simulink model "FDCDC_PSS_40msdelay_Github"  (R2016a)
settings: Solver=ode23t  StartTime=0  StopTime=10  MaxStep=1e-1  RelTol=1e-3
undefined symbols (not defined in the file): D1, delayM2, Delta
libraries: powerlib x29, sps_avr x3, truetime x3, fuzblock x1, spsExcitationSystemModel x1
settings Model: Creator=Administrator  LastModifiedBy=85323
settings SolverCC: SolverResetMethod=Robust
settings DataIOCC: LimitDataPoints=on  SaveFormat=Array
settings HardwareCC: ProdBitPerPointer=32  ProdLargestAtomicFloat=None  ProdIntDivRoundTo=Undefined  ProdEndianess=Unspecified  ProdWordSize=32  ProdHWDeviceType=32-bit Generic
settings ModelReferenceCC: PropagateSignalLabelsOutOfModel=off
settings ConfigComp: CovModelRefEnable=Off

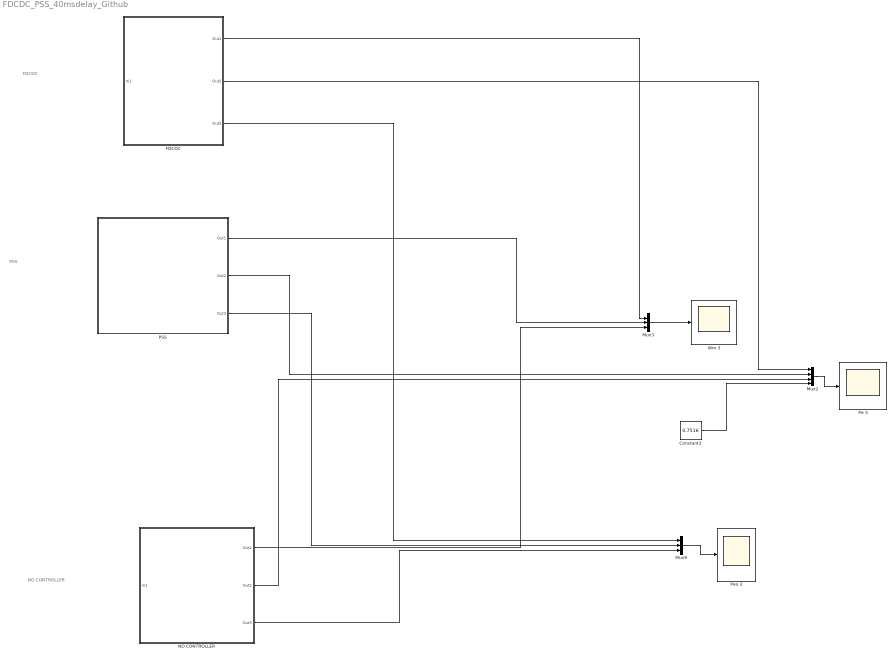
== system FDCDC_PSS_40msdelay_Github ==
  note: PSS
  note: NO
      | CONTROLLER
  note: FDCDC
  Constant3 : Constant  Value=0.7516
  FDCDC : Subsystem
  Mux2 : Mux
  Mux3 : Mux  Inputs=3
  Mux9 : Mux  Inputs=3
  NO CONTROLLER : Subsystem
  PSS : Subsystem
  Pe 3 : Scope
  Peo 3 : Scope
  Wm 3 : Scope
  wires:
  Mux9/1 -> Peo 3/1
  Mux3/1 -> Wm 3/1
  Mux2/1 -> Pe 3/1
  FDCDC/1(Out1) -> Mux3/1
  FDCDC/2(Out2) -> Mux2/1
  FDCDC/3(Out3) -> Mux9/1
  PSS/1(Out1) -> Mux3/2
  PSS/2(Out2) -> Mux2/2
  PSS/3(Out3) -> Mux9/2
  NO CONTROLLER/1(Out1) -> Mux3/3
  NO CONTROLLER/2(Out2) -> Mux2/3
  NO CONTROLLER/3(Out3) -> Mux9/3
  Constant3/1 -> Mux2/4

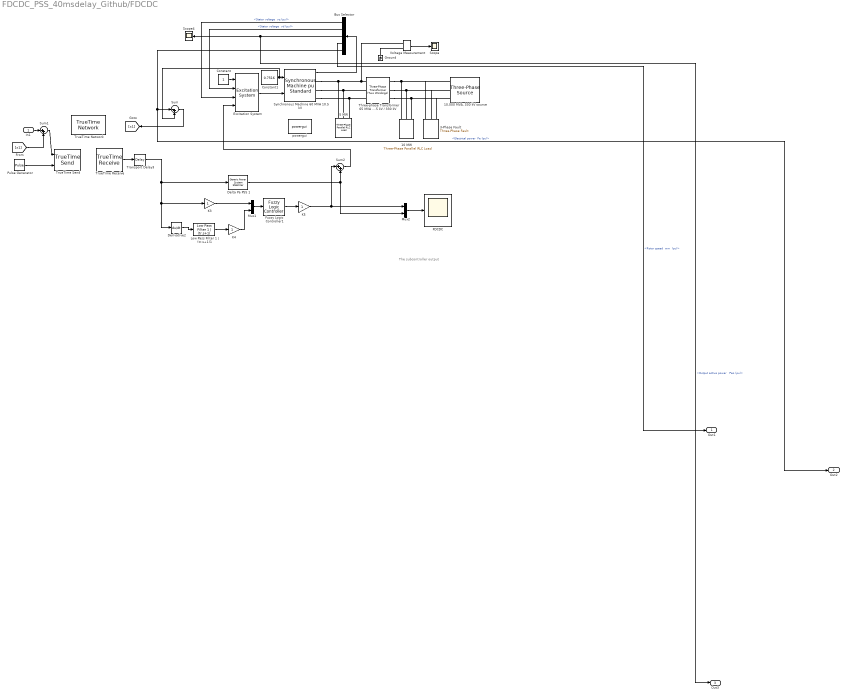
== system FDCDC_PSS_40msdelay_Github/FDCDC ==
  note: The subcontroller output
  In1 : Inport
  10 MW : powerlib/Elements/Three-Phase Parallel RLC Load  LConnTagsString=A|B|C  Configuration=Y (grounded)  NominalVoltage=230e3  Vabc=[1e3 1e3 1e3]  Vabcp=[1e3 1e3 1e3]  NominalFrequency=60  UnbalancedPower=off  ActivePower=10000000  InductivePower=0  CapacitivePower=0  Pabc=[10e3 9e3 11e3]  QLabc=[100 90 110]  QCabc=[100 90 110]  Pabcp=[10e3 9e3 11e3]  QLabcp=[100 90 110]  QCabcp=[100 90 110]  Measurements=None  LoadType=constant Z
  "10,000 MVA, 330 kV source" : powerlib/Electrical Sources/Three-Phase Source  InternalConnection=Yg  VoltagePhases=off  Voltage=(330000)*1.00006  PhaseAngle=-0.77547  Voltage_phases=[25e3 25e3 25e3]/sqrt(3)  PhaseAngles_phases=[0 -120 +120]  Frequency=50  NonIdealSource=on  SpecifyImpedance=on  Resistance=0.529  Inductance=0.0140  ShortCircuitLevel=10000e6  BaseVoltage=230e3  XRratio=10  BusType=swing  Pref=0  Qref=0  Prefabc=[10e3, 10e3, 10e3]  Qrefabc=[0, 0, 0]  Qmin=-Inf  Qmax=Inf
  3-Phase Fault : powerlib/Elements/Three-Phase Fault  InitialStates=0  FaultA=on  FaultB=on  FaultC=on  GroundFault=on  SwitchTimes=[ 2 2.2]  External=off  SwitchStatus=NaN  FaultResistance=1e-3  GroundResistance=1e-3  SnubberResistance=inf  SnubberCapacitance=inf  Measurements=None
  5 MW : powerlib/Elements/Three-Phase Parallel RLC Load  LConnTagsString=A|B|C  Configuration=Y (grounded)  NominalVoltage=13.8e3  Vabc=[1e3 1e3 1e3]  Vabcp=[1e3 1e3 1e3]  NominalFrequency=60  UnbalancedPower=off  ActivePower=5000000  InductivePower=0  CapacitivePower=0  Pabc=[10e3 9e3 11e3]  QLabc=[100 90 110]  QCabc=[100 90 110]  Pabcp=[10e3 9e3 11e3]  QLabcp=[100 90 110]  QCabcp=[100 90 110]  Measurements=None  LoadType=constant Z
  Bus Selector : BusSelector  OutputSignals="dq0 components.Stator voltage  vq (pu),dq0 components.Stator voltage  vd (pu),Output active power   Peo (pu),Mechanical.Rotor speed  wm  (pu),Mechanical.Electrical power  Pe (pu)"
  Constant : Constant
  Constant1 : Constant  Value=0.7516
  Delta Pa PSS 1 : powerlib/Machines/Generic Power System Stabilizer  Tsensor=15e-3  K=2.5*1.25  Twashout=1  Tleadlag1=[60e-3 1]  Tleadlag2=[0 0]  VSlimits=[-1 1]  Vinit=0  Plot_On=off  MagdB_On=off  FreqRange=logspace(-2,2,500)
  Derivative2 : Derivative
  Excitation System : sps_avr/Excitation System  tr=20e-3  reg=[ 300, 0.001 ]  exc=[ 1, 0 ]  tgr=[ 0, 0 ]  damp=[ 0.001, 0.1 ]  sat=[ 0, 0 ]  lim=[ -11.5, 11.5, 0 ]  v0=[1,1.29071]
  FDCDC : Scope
  Fuzzy Logic Controller1 : fuzblock/Fuzzy Logic  Controller  fis=[delayM2]
  Ground : powerlib/Elements/Ground  LConnTagsString=a
  K3 : Gain
  K4 : Gain
  K5 : Gain
  Low Pass Filter 1 | (tr.s+1)1 : spsExcitationSystemModel/Continuous/Low Pass Filter 1 | (tr.s+1)  N=1  D=[0.2 1]  Y0=0  U0=0
  Mux1 : Mux  Inputs=2
  Mux2 : Mux  Inputs=2
  Pulse Generator : DiscretePulseGenerator  PulseType=Time based  Period=0.01  PulseWidth=80
  Scope : Scope
  Scope4 : Scope
  Sum : Sum  Inputs=|-+
  Sum1 : Sum  Inputs=|++
  Sum2 : Sum  Inputs=|++
  Synchronous Machine 60 MVA 10.5 kV : powerlib/Machines/Synchronous Machine pu Standard  PresetModel=No  MechanicalLoad=Mechanical power Pm  ShowDetailedParameters=on  RotorType=Salient-pole  Units=per unit standard parameters  MeasurementBus=off  NominalParameters="[ 60E6  10500   50 ]"  Reactances1=[ 31 32 33 34 35 36 37 ]  Reactances2=[ 1.305, 0.296, 0.252, 0.474, 0.243, 0.18 ]  dAxisTimeConstants=Short-circuit  qAxisTimeConstants=Open-circuit  TimeConstants1=[]  TimeConstants2=[]  TimeConstants3=[]  TimeConstants4=[]  TimeConstants5=[ 1.01, 0.053, 0.1 ]  TimeConstants6=[]  TimeConstants7=[]  TimeConstants8=[]  StatorResistance=2.8544e-3  Mechanical=[ 3.2 0 2]  PolePairs=2  InitialConditions=[0 -94.2826 0.750185 0.750185 0.750185 -24.943 -144.943 95.057 1.29071]  SetSaturation=off  Saturation=[0.6404,0.7127,0.8441,0.9214,0.9956,1.082,1.19,1.316,1.457;0.7,0.7698,0.8872,0.9466,0.9969,1.046,1.1,1.151,1.201]  LoadFlowParameters=[1 150000000 0 0]  TsPowergui=0  TsBlock=-1  IterativeModel=Trapezoidal non iterative  IterativeDiscreteModel=Trapezoidal non iterative  BusType=PV  Pref=150000000  Qref=0  Qmin=-Inf  Qmax=Inf  PLF=0  QLF=0
      settings: AttributesFormatString=\n\n
  Three-phase Transformer 65 MVA 10.5 kV / 330 kV : powerlib/Elements/Three-Phase Transformer (Two Windings)  Winding1Connection=Delta (D1)  Winding2Connection=Yg  CoreType=Three single-phase transformers  SetSaturation=off  Hysteresis=off  DataFile='hysteresis'  SetInitialFlux=off  Measurements=None  UNITS=pu  NominalPower=[ 65e6 50 ]  Winding1="[ 10.5e3 0.0027  0.08]"  Winding2=[ 330e3 0.0027 0.08]  Rm=500  Lm=500  L0=0.5  Saturation="[ 0,0  ;  0.005,1.2  ;  1.0,1.4 ]"  InitialFluxes=[ 0.8 , -0.8 , 0.7 ]  MoreParameters=off  BreakLoop=off  DataType=off  TransfoNumber=0
  Transport Delay3 : TransportDelay  DelayTime=0.04
  TrueTime Network : truetime/TrueTime Network  nwtype=CSMA/CD (Ethernet)  nwnbr=1  nnodes=1  rate=10000000  minsize=512  lossprob=0  seed=0  bandwidths=[0.5 0.5]  slotsize=512  schedule=[1 1 2]  memsize=80000  buftype=Common buffer  overflow=Retransmit  dynSchedule=0  miniSlotSize=0  NIT=0  QSortMode=FIFO  sync=0  irtSchedule=0  nrtLength=0  nodeGraph=0  scheduleoutput=off
  TrueTime Receive : truetime/TrueTime Receive  nwnbr=1  receiver=1  outdim=1  triggeroutput=off  senderoutput=off  lengthoutput=off  priorityoutput=off  timestampoutput=off  signalpoweroutput=off  msgIDoutput=off
  TrueTime Send : truetime/TrueTime Send  trigger=falling  nwnbr=1  sender=1  indim=1  recsource=internal  receiver=1  lengthsource=internal  length=1000  priosource=internal  prio=1  msgIDsource=internal  msgID=0  dynamicSegment=dynamic
  Voltage Measurement : powerlib/Measurements/Voltage Measurement  PhasorSimulation=off  OutputType=Complex  PSBequivalent=0
  powergui : powerlib/powergui  Priority=1  SimulationMode=Continuous  SolverType=Tustin/Backward Euler (TBE)  SampleTime=1e-6  frequency=60  SPID=off  DisableSnubberDevices=off  DisableRonSwitches=off  DisableVfSwitches=off  SwTol=0  DisplayEquations=off  Interpol=off  ExternalGateDelay=off  methode=off  Ts=100  FunctionMessages=off  echomessages=off  HookPort=off  EnableUseOfTLC=off  x0status=blocks  frequencyindice=50  Pbase=100e6  ErrMax=1e-4  Iterations=50  UnitsV=kV  UnitsW=MW  buscounter=0  RestoreLinks=warning  ResistiveCurrentMeasurement=off  Frange=[0:2:500]  Ylog=off  Xlog=on  ShowGrid=off  save=off  variable=ZData  structure=0  ZoomFFT=off  StartTime=0.0  cycles=1  DisplayStyle=1  fundamental=60  FreqAxis=off  MaxFrequency=1000  frequencyindicesteady=1  RmsSteady=1  display=off
  Out1 : Outport
  Out2 : Outport  Port=2
  Out3 : Outport  Port=3
  wires:
  In1/1 -> Sum1/1
  Sum1/1 -> TrueTime Send/1
  Bus Selector/1 -> Excitation System/3  "<Stator voltage  vq (pu)>"
  Pulse Generator/1 -> TrueTime Send/2
  [x1] -> Sum1/2
  Synchronous Machine 60 MVA 10.5 kV/1 -> Bus Selector/1
  Constant/1 -> Excitation System/1
  Bus Selector/3 -> Out3/1, Scope4/1  "<Output active power   Peo (pu)>"
  Bus Selector/5 -> Out2/1, Sum/1  "<Electrical power  Pe (pu)>"
  Voltage Measurement/1 -> Scope/1
  Mux1/1 -> Fuzzy Logic Controller1/1
  K4/1 -> Mux1/2
  Sum/1 -> [x1]
  Derivative2/1 -> Low Pass Filter 1 | (tr.s+1)1/1
  Sum2/1 -> Excitation System/4
  TrueTime Receive/1 -> Transport Delay3/1
  Fuzzy Logic Controller1/1 -> K5/1
  Constant1/1 -> Sum/2, Synchronous Machine 60 MVA 10.5 kV/1
  K3/1 -> Mux1/1
  K5/1 -> Sum2/1, Mux2/1
  Low Pass Filter 1 | (tr.s+1)1/1 -> K4/1
  Transport Delay3/1 -> Delta Pa PSS 1/1, K3/1, Derivative2/1
  Bus Selector/2 -> Excitation System/2  "<Stator voltage  vd (pu)>"
  Bus Selector/4 -> Out1/1  "<Rotor speed  wm  (pu)>"
  Excitation System/1 -> Synchronous Machine 60 MVA 10.5 kV/2
  Delta Pa PSS 1/1 -> Mux2/2, Sum2/2
  Mux2/1 -> FDCDC/1
  connections:
  Voltage Measurement/LConn2 -- Ground/LConn1
  Synchronous Machine 60 MVA 10.5 kV/RConn3 -- Three-phase Transformer 65 MVA 10.5 kV / 330 kV/LConn3 -- 5 MW/LConn3
  Synchronous Machine 60 MVA 10.5 kV/RConn2 -- Three-phase Transformer 65 MVA 10.5 kV / 330 kV/LConn2 -- 5 MW/LConn2
  Three-phase Transformer 65 MVA 10.5 kV / 330 kV/RConn3 -- "10,000 MVA, 330 kV source"/RConn3 -- 3-Phase Fault/LConn3 -- 10 MW/LConn3
  Three-phase Transformer 65 MVA 10.5 kV / 330 kV/RConn1 -- "10,000 MVA, 330 kV source"/RConn1 -- 3-Phase Fault/LConn1 -- 10 MW/LConn1
  Voltage Measurement/LConn1 -- Three-phase Transformer 65 MVA 10.5 kV / 330 kV/LConn1 -- Synchronous Machine 60 MVA 10.5 kV/RConn1 -- 5 MW/LConn1
  Three-phase Transformer 65 MVA 10.5 kV / 330 kV/RConn2 -- "10,000 MVA, 330 kV source"/RConn2 -- 3-Phase Fault/LConn2 -- 10 MW/LConn2

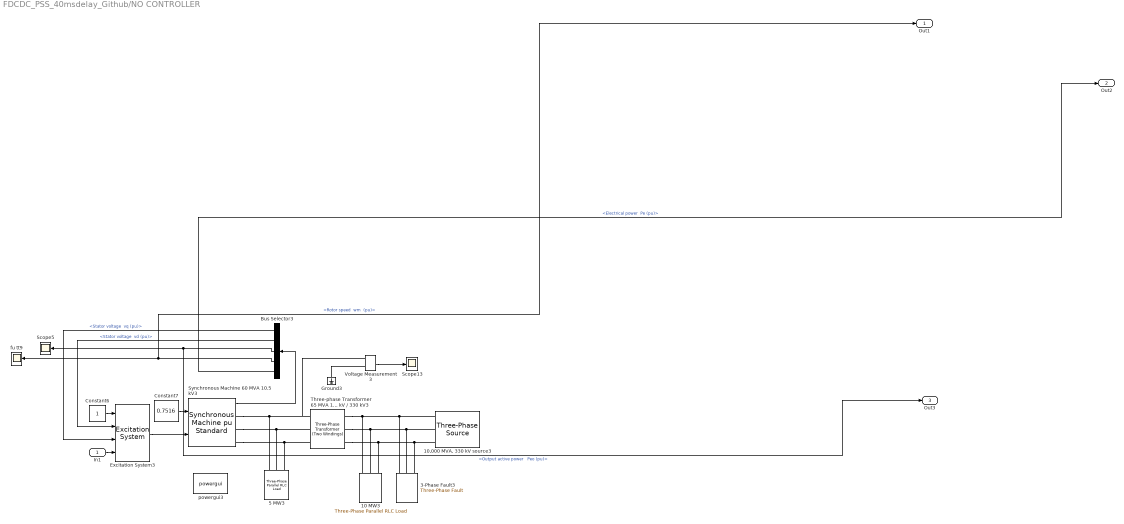
== system FDCDC_PSS_40msdelay_Github/NO CONTROLLER ==
  In1 : Inport
  10 MW3 : powerlib/Elements/Three-Phase Parallel RLC Load  LConnTagsString=A|B|C  Configuration=Y (grounded)  NominalVoltage=230e3  Vabc=[1e3 1e3 1e3]  Vabcp=[1e3 1e3 1e3]  NominalFrequency=60  UnbalancedPower=off  ActivePower=10000000  InductivePower=0  CapacitivePower=0  Pabc=[10e3 9e3 11e3]  QLabc=[100 90 110]  QCabc=[100 90 110]  Pabcp=[10e3 9e3 11e3]  QLabcp=[100 90 110]  QCabcp=[100 90 110]  Measurements=None  LoadType=constant Z
  "10,000 MVA, 330 kV source3" : powerlib/Electrical Sources/Three-Phase Source  InternalConnection=Yg  VoltagePhases=off  Voltage=(330000)*1.00006  PhaseAngle=-0.77547  Voltage_phases=[25e3 25e3 25e3]/sqrt(3)  PhaseAngles_phases=[0 -120 +120]  Frequency=50  NonIdealSource=on  SpecifyImpedance=on  Resistance=0.529  Inductance=0.0140  ShortCircuitLevel=10000e6  BaseVoltage=230e3  XRratio=10  BusType=swing  Pref=0  Qref=0  Prefabc=[10e3, 10e3, 10e3]  Qrefabc=[0, 0, 0]  Qmin=-Inf  Qmax=Inf
  3-Phase Fault3 : powerlib/Elements/Three-Phase Fault  InitialStates=0  FaultA=on  FaultB=on  FaultC=on  GroundFault=on  SwitchTimes=[2 2.2]  External=off  SwitchStatus=NaN  FaultResistance=1e-3  GroundResistance=1e-3  SnubberResistance=inf  SnubberCapacitance=inf  Measurements=None
  5 MW3 : powerlib/Elements/Three-Phase Parallel RLC Load  LConnTagsString=A|B|C  Configuration=Y (grounded)  NominalVoltage=13.8e3  Vabc=[1e3 1e3 1e3]  Vabcp=[1e3 1e3 1e3]  NominalFrequency=60  UnbalancedPower=off  ActivePower=5000000  InductivePower=0  CapacitivePower=0  Pabc=[10e3 9e3 11e3]  QLabc=[100 90 110]  QCabc=[100 90 110]  Pabcp=[10e3 9e3 11e3]  QLabcp=[100 90 110]  QCabcp=[100 90 110]  Measurements=None  LoadType=constant Z
  Bus Selector3 : BusSelector  OutputSignals="dq0 components.Stator voltage  vq (pu),dq0 components.Stator voltage  vd (pu),Output active power   Peo (pu),Mechanical.Rotor speed  wm  (pu),Mechanical.Electrical power  Pe (pu)"
  Constant6 : Constant
  Constant7 : Constant  Value=0.7516
  Excitation System3 : sps_avr/Excitation System  tr=20e-3  reg=[ 300, 0.001 ]  exc=[ 1, 0 ]  tgr=[ 0, 0 ]  damp=[ 0.001, 0.1 ]  sat=[ 0, 0 ]  lim=[ -11.5, 11.5, 0 ]  v0=[1,1.29071]
  Ground3 : powerlib/Elements/Ground  LConnTagsString=a
  Scope13 : Scope
  Scope5 : Scope
  Synchronous Machine 60 MVA 10.5 kV3 : powerlib/Machines/Synchronous Machine pu Standard  PresetModel=No  MechanicalLoad=Mechanical power Pm  ShowDetailedParameters=on  RotorType=Salient-pole  Units=per unit standard parameters  MeasurementBus=off  NominalParameters="[ 60E6  10500   50 ]"  Reactances1=[ 31 32 33 34 35 36 37 ]  Reactances2=[ 1.305, 0.296, 0.252, 0.474, 0.243, 0.18 ]  dAxisTimeConstants=Short-circuit  qAxisTimeConstants=Open-circuit  TimeConstants1=[]  TimeConstants2=[]  TimeConstants3=[]  TimeConstants4=[]  TimeConstants5=[ 1.01, 0.053, 0.1 ]  TimeConstants6=[]  TimeConstants7=[]  TimeConstants8=[]  StatorResistance=2.8544e-3  Mechanical=[ 3.2 0 2]  PolePairs=2  InitialConditions=[0 -94.2826 0.750185 0.750185 0.750185 -24.943 -144.943 95.057 1.29071]  SetSaturation=off  Saturation=[0.6404,0.7127,0.8441,0.9214,0.9956,1.082,1.19,1.316,1.457;0.7,0.7698,0.8872,0.9466,0.9969,1.046,1.1,1.151,1.201]  LoadFlowParameters=[1 150000000 0 0]  TsPowergui=0  TsBlock=-1  IterativeModel=Trapezoidal non iterative  IterativeDiscreteModel=Trapezoidal non iterative  BusType=PV  Pref=150000000  Qref=0  Qmin=-Inf  Qmax=Inf  PLF=0  QLF=0
      settings: AttributesFormatString=\n\n
  Three-phase Transformer 65 MVA 10.5 kV / 330 kV3 : powerlib/Elements/Three-Phase Transformer (Two Windings)  Winding1Connection=Delta (D1)  Winding2Connection=Yg  CoreType=Three single-phase transformers  SetSaturation=off  Hysteresis=off  DataFile='hysteresis'  SetInitialFlux=off  Measurements=None  UNITS=pu  NominalPower=[ 65e6 50 ]  Winding1="[ 10.5e3 0.0027  0.08]"  Winding2=[ 330e3 0.0027 0.08]  Rm=500  Lm=500  L0=0.5  Saturation="[ 0,0  ;  0.005,1.2  ;  1.0,1.4 ]"  InitialFluxes=[ 0.8 , -0.8 , 0.7 ]  MoreParameters=off  BreakLoop=off  DataType=off  TransfoNumber=0
  Voltage Measurement3 : powerlib/Measurements/Voltage Measurement  PhasorSimulation=off  OutputType=Complex  PSBequivalent=0
  fu tt9 : Scope
  powergui3 : powerlib/powergui  Priority=1  SimulationMode=Continuous  SolverType=Tustin/Backward Euler (TBE)  SampleTime=1e-6  frequency=60  SPID=off  DisableSnubberDevices=off  DisableRonSwitches=off  DisableVfSwitches=off  SwTol=0  DisplayEquations=off  Interpol=off  ExternalGateDelay=off  methode=off  Ts=100  FunctionMessages=off  echomessages=off  HookPort=off  EnableUseOfTLC=off  x0status=blocks  frequencyindice=50  Pbase=100e6  ErrMax=1e-4  Iterations=50  UnitsV=kV  UnitsW=MW  buscounter=0  RestoreLinks=warning  ResistiveCurrentMeasurement=off  Frange=[0:2:500]  Ylog=off  Xlog=on  ShowGrid=off  save=off  variable=ZData  structure=0  ZoomFFT=off  StartTime=0.0  cycles=1  DisplayStyle=1  fundamental=60  FreqAxis=off  MaxFrequency=1000  frequencyindicesteady=1  RmsSteady=1  display=off
  Out1 : Outport
  Out2 : Outport  Port=2
  Out3 : Outport  Port=3
  wires:
  Bus Selector3/5 -> Out2/1  "<Electrical power  Pe (pu)>"
  Bus Selector3/3 -> Out3/1, Scope5/1  "<Output active power   Peo (pu)>"
  Constant7/1 -> Synchronous Machine 60 MVA 10.5 kV3/1
  Synchronous Machine 60 MVA 10.5 kV3/1 -> Bus Selector3/1
  Voltage Measurement3/1 -> Scope13/1
  Bus Selector3/4 -> Out1/1, fu tt9/1  "<Rotor speed  wm  (pu)>"
  Bus Selector3/2 -> Excitation System3/2  "<Stator voltage  vd (pu)>"
  Constant6/1 -> Excitation System3/1
  Excitation System3/1 -> Synchronous Machine 60 MVA 10.5 kV3/2
  Bus Selector3/1 -> Excitation System3/3  "<Stator voltage  vq (pu)>"
  In1/1 -> Excitation System3/4
  connections:
  Three-phase Transformer 65 MVA 10.5 kV / 330 kV3/LConn3 -- 5 MW3/LConn3 -- Synchronous Machine 60 MVA 10.5 kV3/RConn3
  3-Phase Fault3/LConn3 -- "10,000 MVA, 330 kV source3"/RConn3 -- 10 MW3/LConn3 -- Three-phase Transformer 65 MVA 10.5 kV / 330 kV3/RConn3
  3-Phase Fault3/LConn2 -- "10,000 MVA, 330 kV source3"/RConn2 -- 10 MW3/LConn2 -- Three-phase Transformer 65 MVA 10.5 kV / 330 kV3/RConn2
  3-Phase Fault3/LConn1 -- "10,000 MVA, 330 kV source3"/RConn1 -- 10 MW3/LConn1 -- Three-phase Transformer 65 MVA 10.5 kV / 330 kV3/RConn1
  Three-phase Transformer 65 MVA 10.5 kV / 330 kV3/LConn2 -- 5 MW3/LConn2 -- Synchronous Machine 60 MVA 10.5 kV3/RConn2
  Voltage Measurement3/LConn2 -- Ground3/LConn1
  5 MW3/LConn1 -- Synchronous Machine 60 MVA 10.5 kV3/RConn1 -- Three-phase Transformer 65 MVA 10.5 kV / 330 kV3/LConn1 -- Voltage Measurement3/LConn1

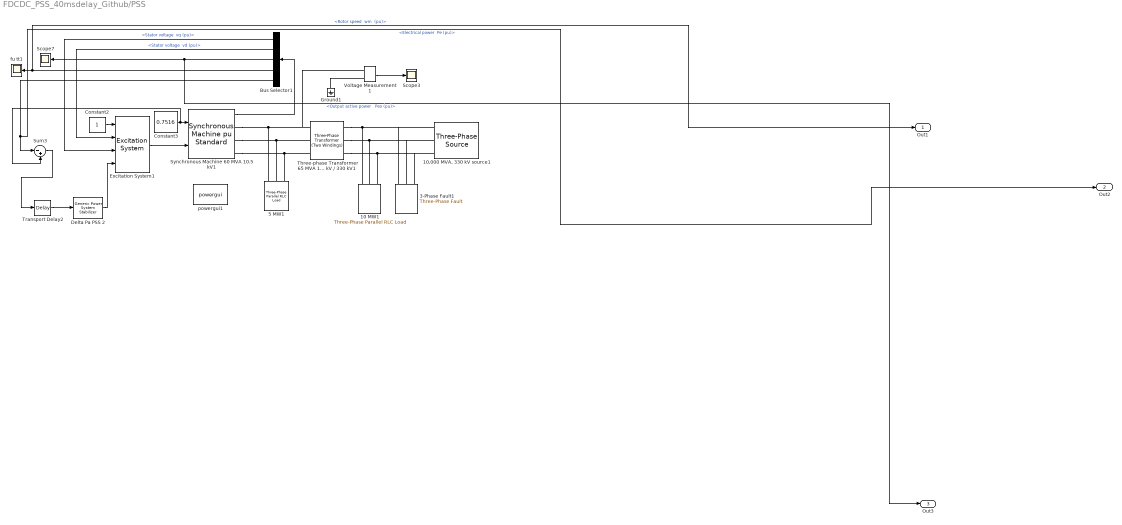
== system FDCDC_PSS_40msdelay_Github/PSS ==
  10 MW1 : powerlib/Elements/Three-Phase Parallel RLC Load  LConnTagsString=A|B|C  Configuration=Y (grounded)  NominalVoltage=230e3  Vabc=[1e3 1e3 1e3]  Vabcp=[1e3 1e3 1e3]  NominalFrequency=60  UnbalancedPower=off  ActivePower=10000000  InductivePower=0  CapacitivePower=0  Pabc=[10e3 9e3 11e3]  QLabc=[100 90 110]  QCabc=[100 90 110]  Pabcp=[10e3 9e3 11e3]  QLabcp=[100 90 110]  QCabcp=[100 90 110]  Measurements=None  LoadType=constant Z
  "10,000 MVA, 330 kV source1" : powerlib/Electrical Sources/Three-Phase Source  InternalConnection=Yg  VoltagePhases=off  Voltage=(330000)*1.00006  PhaseAngle=-0.77547  Voltage_phases=[25e3 25e3 25e3]/sqrt(3)  PhaseAngles_phases=[0 -120 +120]  Frequency=50  NonIdealSource=on  SpecifyImpedance=on  Resistance=0.529  Inductance=0.0140  ShortCircuitLevel=10000e6  BaseVoltage=230e3  XRratio=10  BusType=swing  Pref=0  Qref=0  Prefabc=[10e3, 10e3, 10e3]  Qrefabc=[0, 0, 0]  Qmin=-Inf  Qmax=Inf
  3-Phase Fault1 : powerlib/Elements/Three-Phase Fault  InitialStates=0  FaultA=on  FaultB=on  FaultC=on  GroundFault=on  SwitchTimes=[ 2 2.2]  External=off  SwitchStatus=NaN  FaultResistance=1e-3  GroundResistance=1e-3  SnubberResistance=inf  SnubberCapacitance=inf  Measurements=None
  5 MW1 : powerlib/Elements/Three-Phase Parallel RLC Load  LConnTagsString=A|B|C  Configuration=Y (grounded)  NominalVoltage=13.8e3  Vabc=[1e3 1e3 1e3]  Vabcp=[1e3 1e3 1e3]  NominalFrequency=60  UnbalancedPower=off  ActivePower=5000000  InductivePower=0  CapacitivePower=0  Pabc=[10e3 9e3 11e3]  QLabc=[100 90 110]  QCabc=[100 90 110]  Pabcp=[10e3 9e3 11e3]  QLabcp=[100 90 110]  QCabcp=[100 90 110]  Measurements=None  LoadType=constant Z
  Bus Selector1 : BusSelector  OutputSignals="dq0 components.Stator voltage  vq (pu),dq0 components.Stator voltage  vd (pu),Output active power   Peo (pu),Mechanical.Rotor speed  wm  (pu),Mechanical.Electrical power  Pe (pu)"
  Constant2 : Constant
  Constant3 : Constant  Value=0.7516
  Delta Pa PSS 2 : powerlib/Machines/Generic Power System Stabilizer  Tsensor=15e-3  K=2.5*1.25  Twashout=1  Tleadlag1=[60e-3 1]  Tleadlag2=[0 0]  VSlimits=[-1 1]  Vinit=0  Plot_On=off  MagdB_On=off  FreqRange=logspace(-2,2,500)
  Excitation System1 : sps_avr/Excitation System  tr=20e-3  reg=[ 300, 0.001 ]  exc=[ 1, 0 ]  tgr=[ 0, 0 ]  damp=[ 0.001, 0.1 ]  sat=[ 0, 0 ]  lim=[ -11.5, 11.5, 0 ]  v0=[1,1.29071]
  Ground1 : powerlib/Elements/Ground  LConnTagsString=a
  Scope3 : Scope
  Scope7 : Scope
  Sum3 : Sum  Inputs=|-+
  Synchronous Machine 60 MVA 10.5 kV1 : powerlib/Machines/Synchronous Machine pu Standard  PresetModel=No  MechanicalLoad=Mechanical power Pm  ShowDetailedParameters=on  RotorType=Salient-pole  Units=per unit standard parameters  MeasurementBus=off  NominalParameters="[ 60E6  10500   50 ]"  Reactances1=[ 31 32 33 34 35 36 37 ]  Reactances2=[ 1.305, 0.296, 0.252, 0.474, 0.243, 0.18 ]  dAxisTimeConstants=Short-circuit  qAxisTimeConstants=Open-circuit  TimeConstants1=[]  TimeConstants2=[]  TimeConstants3=[]  TimeConstants4=[]  TimeConstants5=[ 1.01, 0.053, 0.1 ]  TimeConstants6=[]  TimeConstants7=[]  TimeConstants8=[]  StatorResistance=2.8544e-3  Mechanical=[ 3.2 0 2]  PolePairs=2  InitialConditions=[0 -94.2826 0.750185 0.750185 0.750185 -24.943 -144.943 95.057 1.29071]  SetSaturation=off  Saturation=[0.6404,0.7127,0.8441,0.9214,0.9956,1.082,1.19,1.316,1.457;0.7,0.7698,0.8872,0.9466,0.9969,1.046,1.1,1.151,1.201]  LoadFlowParameters=[1 150000000 0 0]  TsPowergui=0  TsBlock=-1  IterativeModel=Trapezoidal non iterative  IterativeDiscreteModel=Trapezoidal non iterative  BusType=PV  Pref=150000000  Qref=0  Qmin=-Inf  Qmax=Inf  PLF=0  QLF=0
      settings: AttributesFormatString=\n\n
  Three-phase Transformer 65 MVA 10.5 kV / 330 kV1 : powerlib/Elements/Three-Phase Transformer (Two Windings)  Winding1Connection=Delta (D1)  Winding2Connection=Yg  CoreType=Three single-phase transformers  SetSaturation=off  Hysteresis=off  DataFile='hysteresis'  SetInitialFlux=off  Measurements=None  UNITS=pu  NominalPower=[ 65e6 50 ]  Winding1="[ 10.5e3 0.0027  0.08]"  Winding2=[ 330e3 0.0027 0.08]  Rm=500  Lm=500  L0=0.5  Saturation="[ 0,0  ;  0.005,1.2  ;  1.0,1.4 ]"  InitialFluxes=[ 0.8 , -0.8 , 0.7 ]  MoreParameters=off  BreakLoop=off  DataType=off  TransfoNumber=0
  Transport Delay2 : TransportDelay  DelayTime=0.04
  Voltage Measurement1 : powerlib/Measurements/Voltage Measurement  PhasorSimulation=off  OutputType=Complex  PSBequivalent=0
  fu tt1 : Scope
  powergui1 : powerlib/powergui  Priority=1  SimulationMode=Continuous  SolverType=Tustin/Backward Euler (TBE)  SampleTime=1e-6  frequency=60  SPID=off  DisableSnubberDevices=off  DisableRonSwitches=off  DisableVfSwitches=off  SwTol=0  DisplayEquations=off  Interpol=off  ExternalGateDelay=off  methode=off  Ts=100  FunctionMessages=off  echomessages=off  HookPort=off  EnableUseOfTLC=off  x0status=blocks  frequencyindice=50  Pbase=100e6  ErrMax=1e-4  Iterations=50  UnitsV=kV  UnitsW=MW  buscounter=0  RestoreLinks=warning  ResistiveCurrentMeasurement=off  Frange=[0:2:500]  Ylog=off  Xlog=on  ShowGrid=off  save=off  variable=ZData  structure=0  ZoomFFT=off  StartTime=0.0  cycles=1  DisplayStyle=1  fundamental=60  FreqAxis=off  MaxFrequency=1000  frequencyindicesteady=1  RmsSteady=1  display=off
  Out1 : Outport
  Out2 : Outport  Port=2
  Out3 : Outport  Port=3
  wires:
  Bus Selector1/1 -> Excitation System1/3  "<Stator voltage  vq (pu)>"
  Synchronous Machine 60 MVA 10.5 kV1/1 -> Bus Selector1/1
  Sum3/1 -> Transport Delay2/1
  Bus Selector1/2 -> Excitation System1/2  "<Stator voltage  vd (pu)>"
  Excitation System1/1 -> Synchronous Machine 60 MVA 10.5 kV1/2
  Transport Delay2/1 -> Delta Pa PSS 2/1
  Bus Selector1/5 -> Out2/1, Sum3/1  "<Electrical power  Pe (pu)>"
  Delta Pa PSS 2/1 -> Excitation System1/4
  Bus Selector1/4 -> Out1/1, fu tt1/1  "<Rotor speed  wm  (pu)>"
  Constant2/1 -> Excitation System1/1
  Constant3/1 -> Sum3/2, Synchronous Machine 60 MVA 10.5 kV1/1
  Bus Selector1/3 -> Out3/1, Scope7/1  "<Output active power   Peo (pu)>"
  Voltage Measurement1/1 -> Scope3/1
  connections:
  5 MW1/LConn2 -- Synchronous Machine 60 MVA 10.5 kV1/RConn2 -- Three-phase Transformer 65 MVA 10.5 kV / 330 kV1/LConn2
  5 MW1/LConn1 -- Synchronous Machine 60 MVA 10.5 kV1/RConn1 -- Voltage Measurement1/LConn1 -- Three-phase Transformer 65 MVA 10.5 kV / 330 kV1/LConn1
  5 MW1/LConn3 -- Synchronous Machine 60 MVA 10.5 kV1/RConn3 -- Three-phase Transformer 65 MVA 10.5 kV / 330 kV1/LConn3
  10 MW1/LConn1 -- Three-phase Transformer 65 MVA 10.5 kV / 330 kV1/RConn1 -- "10,000 MVA, 330 kV source1"/RConn1 -- 3-Phase Fault1/LConn1
  10 MW1/LConn2 -- Three-phase Transformer 65 MVA 10.5 kV / 330 kV1/RConn2 -- "10,000 MVA, 330 kV source1"/RConn2 -- 3-Phase Fault1/LConn2
  Voltage Measurement1/LConn2 -- Ground1/LConn1
  10 MW1/LConn3 -- Three-phase Transformer 65 MVA 10.5 kV / 330 kV1/RConn3 -- "10,000 MVA, 330 kV source1"/RConn3 -- 3-Phase Fault1/LConn3
